simulink model "Integrated_Model"  (R2023b)
settings: Solver=ode23s  StartTime=0.0  StopTime=120  FixedStep=0.01  RelTol=1e-3
undefined symbols (not defined in the file): A_sm, A_stack, A_VGS_center, cmp, cp_coolant, ctrl, estNcr, eta_hex, eta_M, J_rotor, k_e_M, k_t_M, lambda, M_H2O, M_Nmix, M_O2, m_st_Nmix_init, m_st_O2_init, m_st_vp_init, p_amb, p_init, R_init, R_M, R_Nmix, R_O2, R_vp, RH_amb, T_amb, T_coolant, T_init, tbn, V_sm, V_stack, V_tbn_m, yO2_amb
libraries: slpidlib x5
(part 3 of 3)

== matlab function Integrated_Model/Supply manifold/Nozzle/calc_phi ==
  data: pin input; phi output; pout input; kap input
function phi = fcn(pin,pout,kap)
    pr = pout/pin;
    p_cr = (2/(kap+1))^(kap/(kap-1))*pin;
    % Judge critical pressure
    if pout < p_cr
        tmp_phi = sqrt(kap*(2/(kap+1))^((kap+1)/(kap-1)));
    else
        % Prevent to become minus values
        a = 1-pr^((kap-1)/kap);
        if a < 0
           a = 0;
        end
        tmp_phi = pr^(1/kap)*sqrt(2*kap/(kap-1)*(a));
    end
    phi = tmp_phi;
end

== matlab function Integrated_Model/Simple Compressor/Subsystem/MATLAB Function1 ==
  data: Ts input; psat output
function psat = sat_vp_pressure(Ts)
    P_CONVERT = 0.001;
    C1 = -5.6745359e3;
    C2 = 6.3925247;
    C3 = -9.6778430e-3;
    C4 = 6.2215701e-7;
    C5 = 2.0747825e-9;
    C6 = -9.4840240e-13;
    C7 = 4.1635019;
    N1 = 0.11670521452767e4;
    N2 = -0.72421316703206e6;
    N3 = -0.17073846940092e2;
    N4 = 0.12020824702470e5;
    N5 = -0.32325550322333e7;
    N6 = 0.14915108613530e2;
    N7 = -0.4823265731591e4;
    N8 = 0.40511340542057e6;
    N9 = -0.23855557567849e0;
    N10 = 0.65017534844798e3;
    
    if Ts < 273.15+0.01
        % -100~0.01C//三重点を計算以下は wexler-hyland のシミュレーションプログラム式
        psat = exp(C1 / Ts + C2 + C3 * Ts + C4 * Ts^2 + C5 * Ts^3 + C6 * Ts^4 + C7 * log(Ts)) * P_CONVERT;
    else
        %　~647.096K//臨界温度まで一定とするは IAPWS-IF97 実用国際状態式
        alpha = Ts + N9 / (Ts - N10);
        a2 = alpha * alpha;
        A = a2 + N1 * alpha + N2;
        B = N3 * a2 + N4 * alpha + N5;
        C = N6 * a2 + N7 * alpha + N8;
        psat = (2 * C / (-B + (B * B - 4 * A * C)^0.5))^4 / P_CONVERT;
    end 
    psat = psat*1000; %kPa to Pa
end

== matlab function Integrated_Model/Supply manifold/Subsystem/MATLAB Function ==
  data: Ts input; psat output
function psat = sat_vp_pressure(Ts)
    P_CONVERT = 0.001;
    C1 = -5.6745359e3;
    C2 = 6.3925247;
    C3 = -9.6778430e-3;
    C4 = 6.2215701e-7;
    C5 = 2.0747825e-9;
    C6 = -9.4840240e-13;
    C7 = 4.1635019;
    N1 = 0.11670521452767e4;
    N2 = -0.72421316703206e6;
    N3 = -0.17073846940092e2;
    N4 = 0.12020824702470e5;
    N5 = -0.32325550322333e7;
    N6 = 0.14915108613530e2;
    N7 = -0.4823265731591e4;
    N8 = 0.40511340542057e6;
    N9 = -0.23855557567849e0;
    N10 = 0.65017534844798e3;
    
    if Ts < 273.15+0.01
        % -100~0.01C//三重点を計算以下は wexler-hyland のシミュレーションプログラム式
        psat = exp(C1 / Ts + C2 + C3 * Ts + C4 * Ts^2 + C5 * Ts^3 + C6 * Ts^4 + C7 * log(Ts)) * P_CONVERT;
    else
        %　~647.096K//臨界温度まで一定とするは IAPWS-IF97 実用国際状態式
        alpha = Ts + N9 / (Ts - N10);
        a2 = alpha * alpha;
        A = a2 + N1 * alpha + N2;
        B = N3 * a2 + N4 * alpha + N5;
        C = N6 * a2 + N7 * alpha + N8;
        psat = (2 * C / (-B + (B * B - 4 * A * C)^0.5))^4 / P_CONVERT;
    end 
    psat = psat*1000; %kPa to Pa
end

== matlab function Integrated_Model/Supply manifold/Subsystem/MATLAB Function1 ==
  data: Ts input; psat output
function psat = sat_vp_pressure(Ts)
    P_CONVERT = 0.001;
    C1 = -5.6745359e3;
    C2 = 6.3925247;
    C3 = -9.6778430e-3;
    C4 = 6.2215701e-7;
    C5 = 2.0747825e-9;
    C6 = -9.4840240e-13;
    C7 = 4.1635019;
    N1 = 0.11670521452767e4;
    N2 = -0.72421316703206e6;
    N3 = -0.17073846940092e2;
    N4 = 0.12020824702470e5;
    N5 = -0.32325550322333e7;
    N6 = 0.14915108613530e2;
    N7 = -0.4823265731591e4;
    N8 = 0.40511340542057e6;
    N9 = -0.23855557567849e0;
    N10 = 0.65017534844798e3;
    
    if Ts < 273.15+0.01
        % -100~0.01C//三重点を計算以下は wexler-hyland のシミュレーションプログラム式
        psat = exp(C1 / Ts + C2 + C3 * Ts + C4 * Ts^2 + C5 * Ts^3 + C6 * Ts^4 + C7 * log(Ts)) * P_CONVERT;
    else
        %　~647.096K//臨界温度まで一定とするは IAPWS-IF97 実用国際状態式
        alpha = Ts + N9 / (Ts - N10);
        a2 = alpha * alpha;
        A = a2 + N1 * alpha + N2;
        B = N3 * a2 + N4 * alpha + N5;
        C = N6 * a2 + N7 * alpha + N8;
        psat = (2 * C / (-B + (B * B - 4 * A * C)^0.5))^4 / P_CONVERT;
    end 
    psat = psat*1000; %kPa to Pa
end

== matlab function Integrated_Model/SimpleTurbine/SimpleFlowCalculator(Orifice)/calc_phi ==
  data: pin input; phi output; pout input; kap input
function phi = fcn(pin,pout,kap)
    pr = pout/pin;
    p_cr = (2/(kap+1))^(kap/(kap-1))*pin;
    % Judge critical pressure
    if pout < p_cr
        tmp_phi = sqrt(kap*(2/(kap+1))^((kap+1)/(kap-1)));
    else
        % Prevent to become minus values
        a = 1-pr^((kap-1)/kap);
        if a < 0
           a = 0;
        end
        tmp_phi = pr^(1/kap)*sqrt(2*kap/(kap-1)*(a));
    end
    phi = tmp_phi;
end

== matlab function Integrated_Model/SimpleTurbine/ThermoDynamics ==
  data: Pi input; To output; To_dry output; Po input; Ti input; RHi input; eff_tbn input; RHo output; kap input; cp_air input
function [To,To_dry,RHo] = fcn(Pi,Po,Ti,RHi,eff_tbn,kap,cp_air)

% Physical property
cp_vapor = 1.805;
cp_H2O   = 4.186;

% Calc moist air property
Pwsi = calc_sat_pressure(Ti);   % kPa
Pwi = RHi*Pwsi;             % kPa
Wi = 0.62198*Pwi/(Pi-Pwi);      % kg/kg

% calc adiabatic expansion
To_dry = Ti - eff_tbn*Ti*(1-(Pi/Po)^(-(kap-1)/kap));
ho_dry = calc_entalpy_air(To_dry, cp_air/1000, cp_vapor, Wi, 2501.0);

% 凝縮ジャッジ
Pwo = Pwi/Pi*Po;
Pwso = calc_sat_pressure(To_dry);

if Pwo > Pwso
    % disp("凝縮！");
    % Solve turbine outlet temperature by Newton–Raphson method
    % Solver setting
    iteration = 0;
    delta = 1e-10;
    error_min = 1e-5;
    error = 1;
    max_iteration = 999;
    % Initial state
    To = To_dry;
    RHo = 1;

    while error > error_min && iteration < max_iteration
        Pwso = calc_sat_pressure(To);
        Wo = 0.62198*Pwso/(Po-Pwso);
        ho = calc_entalpy_mix(To, cp_air/1000, cp_vapor, cp_H2O, Wi, Wo, 2501.0);
        fn = ho_dry - ho;
        Pwso_delta = calc_sat_pressure(To+delta);
        Wo_delta = 0.62198*Pwso_delta/(Po-Pwso_delta);
        ho_delta = calc_entalpy_mix(To+delta, cp_air/1000, cp_vapor, cp_H2O, Wi, Wo, 2501.0);
        fn_delta = ho_dry - ho_delta;
        df = (fn_delta-fn)/delta;
        df2 = fn/df;
        To = To - 0.01 * fn/((fn_delta-fn)/delta);
        error = abs(ho_dry - calc_entalpy_mix(To, cp_air/1000, cp_vapor, cp_H2O, Wi, Wo, 2501.0));
        iteration = iteration + 1;
    end
else
    To = To_dry;
    RHo = Pwo/Pwso;
end

end

function F = calc_sat_pressure(Ts)
    P_CONVERT = 0.001;
    C1 = -5.6745359e3;
    C2 = 6.3925247;
    C3 = -9.6778430e-3;
    C4 = 6.2215701e-7;
    C5 = 2.0747825e-9;
    C6 = -9.4840240e-13;
    C7 = 4.1635019;
    N1 = 0.11670521452767e4;
    N2 = -0.72421316703206e6;
    N3 = -0.17073846940092e2;
    N4 = 0.12020824702470e5;
    N5 = -0.32325550322333e7;
    N6 = 0.14915108613530e2;
    N7 = -0.4823265731591e4;
    N8 = 0.40511340542057e6;
    N9 = -0.23855557567849e0;
    N10 = 0.65017534844798e3;
    
    if Ts < 273.15+0.01
        % -100~0.01C//三重点を計算以下は wexler-hyland のシミュレーションプログラム式
        psat = exp(C1 / Ts + C2 + C3 * Ts + C4 * Ts^2 + C5 * Ts^3 + C6 * Ts^4 + C7 * log(Ts)) * P_CONVERT;
    else
        %　~647.096K//臨界温度まで一定とするは IAPWS-IF97 実用国際状態式
        alpha = Ts + N9 / (Ts - N10);
        a2 = alpha * alpha;
        A = a2 + N1 * alpha + N2;
        B = N3 * a2 + N4 * alpha + N5;
        C = N6 * a2 + N7 * alpha + N8;
        psat = (2 * C / (-B + (B * B - 4 * A * C)^0.5))^4 / P_CONVERT;
    end 
    F = psat*1000; %kPa to Pa
end

function F = calc_entalpy_air(T,Cpa,Cpv,W,hg0)
    F = Cpa*T+W*(Cpv*T+hg0);
end

function F = calc_entalpy_mix(T,Cpa,Cpv,Cpw,W1,W2,hg0)
    F = Cpa*T+W2*(Cpv*T+hg0)+(W1-W2)*Cpw*T;
end

== matlab function Integrated_Model/SimpleFCstack/Cathode dynamics/Calc inlet mass flow state/Calc absolute humidity ratio [kg//kgDA]/MATLAB Function1 ==
  data: Ts input; psat output
function psat = sat_vp_pressure(Ts)
    P_CONVERT = 0.001;
    C1 = -5.6745359e3;
    C2 = 6.3925247;
    C3 = -9.6778430e-3;
    C4 = 6.2215701e-7;
    C5 = 2.0747825e-9;
    C6 = -9.4840240e-13;
    C7 = 4.1635019;
    N1 = 0.11670521452767e4;
    N2 = -0.72421316703206e6;
    N3 = -0.17073846940092e2;
    N4 = 0.12020824702470e5;
    N5 = -0.32325550322333e7;
    N6 = 0.14915108613530e2;
    N7 = -0.4823265731591e4;
    N8 = 0.40511340542057e6;
    N9 = -0.23855557567849e0;
    N10 = 0.65017534844798e3;
    
    if Ts < 273.15+0.01
        % -100~0.01C//三重点を計算以下は wexler-hyland のシミュレーションプログラム式
        psat = exp(C1 / Ts + C2 + C3 * Ts + C4 * Ts^2 + C5 * Ts^3 + C6 * Ts^4 + C7 * log(Ts)) * P_CONVERT;
    else
        %　~647.096K//臨界温度まで一定とするは IAPWS-IF97 実用国際状態式
        alpha = Ts + N9 / (Ts - N10);
        a2 = alpha * alpha;
        A = a2 + N1 * alpha + N2;
        B = N3 * a2 + N4 * alpha + N5;
        C = N6 * a2 + N7 * alpha + N8;
        psat = (2 * C / (-B + (B * B - 4 * A * C)^0.5))^4 / P_CONVERT;
    end 
    psat = psat*1000; %kPa to Pa
end

== matlab function Integrated_Model/SimpleFCstack/Cathode dynamics/Calc outlet mass flow state/Calc absolute humidity ratio [kg//kgDA]/MATLAB Function1 ==
  data: Ts input; psat output
function psat = sat_vp_pressure(Ts)
    P_CONVERT = 0.001;
    C1 = -5.6745359e3;
    C2 = 6.3925247;
    C3 = -9.6778430e-3;
    C4 = 6.2215701e-7;
    C5 = 2.0747825e-9;
    C6 = -9.4840240e-13;
    C7 = 4.1635019;
    N1 = 0.11670521452767e4;
    N2 = -0.72421316703206e6;
    N3 = -0.17073846940092e2;
    N4 = 0.12020824702470e5;
    N5 = -0.32325550322333e7;
    N6 = 0.14915108613530e2;
    N7 = -0.4823265731591e4;
    N8 = 0.40511340542057e6;
    N9 = -0.23855557567849e0;
    N10 = 0.65017534844798e3;
    
    if Ts < 273.15+0.01
        % -100~0.01C//三重点を計算以下は wexler-hyland のシミュレーションプログラム式
        psat = exp(C1 / Ts + C2 + C3 * Ts + C4 * Ts^2 + C5 * Ts^3 + C6 * Ts^4 + C7 * log(Ts)) * P_CONVERT;
    else
        %　~647.096K//臨界温度まで一定とするは IAPWS-IF97 実用国際状態式
        alpha = Ts + N9 / (Ts - N10);
        a2 = alpha * alpha;
        A = a2 + N1 * alpha + N2;
        B = N3 * a2 + N4 * alpha + N5;
        C = N6 * a2 + N7 * alpha + N8;
        psat = (2 * C / (-B + (B * B - 4 * A * C)^0.5))^4 / P_CONVERT;
    end 
    psat = psat*1000; %kPa to Pa
end
